simulink model "Week1_problem2"  (R2020b)
settings: Solver=VariableStepAuto  StartTime=0.0  StopTime=100.0  RelTol=1e-3
values from neighbouring files (symbols this model uses):
  b = 50    [parameter_initialize.m]
  k1 = 10    [parameter_initialize.m]
  k2 = 20    [parameter_initialize.m]
  M1 = 100    [parameter_initialize.m]
  M2 = 50    [parameter_initialize.m]
settings Model: Creator=omkar  LastModifiedBy=omkar

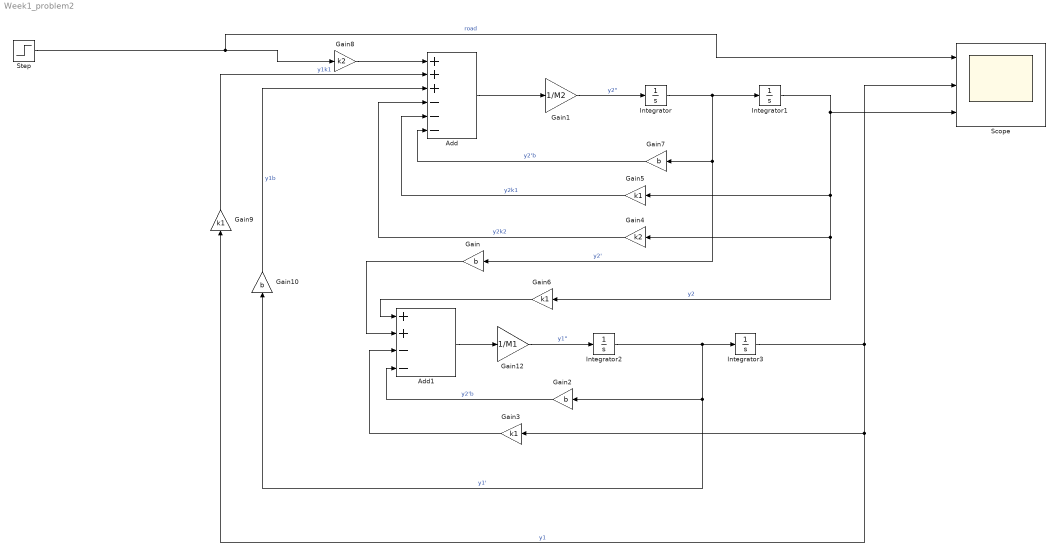
== system Week1_problem2 ==
  Add : Sum  Inputs=+++---
  Add1 : Sum  Inputs=++--
  Gain{,2,7,10} (4 alike) : Gain  Gain=b
  Gain1 : Gain  Gain=1/M2
  Gain12 : Gain  Gain=1/M1
  Gain{3,5..6,9} (4 alike) : Gain  Gain=k1
  Gain4 : Gain  Gain=k2
  Gain8 : Gain  Gain=k2
  Integrator{,1..3} (4 alike) : Integrator
  Scope : Scope  NumInputPorts=3
  Step : Step  SampleTime=0
  wires:
  Add/1 -> Gain1/1
  Gain1/1 -> Integrator/1  "y2\""
  Integrator/1 -> Gain/1, Gain7/1, Integrator1/1  "y2'"
  Gain7/1 -> Add/6  "y2'b"
  Integrator1/1 -> Gain5/1, Gain4/1, Gain6/1, Scope/3  "y2"
  Gain6/1 -> Add1/1
  Gain/1 -> Add1/2
  Add1/1 -> Gain12/1
  Gain12/1 -> Integrator2/1  "y1\""
  Integrator2/1 -> Gain2/1, Gain10/1, Integrator3/1  "y1'"
  Integrator3/1 -> Scope/2, Gain3/1, Gain9/1  "y1"
  Gain2/1 -> Add1/4  "y2'b"
  Gain3/1 -> Add1/3
  Gain5/1 -> Add/5  "y2k1"
  Gain4/1 -> Add/4  "y2k2"
  Gain8/1 -> Add/1
  Gain9/1 -> Add/2  "y1k1"
  Gain10/1 -> Add/3  "y1b"
  Step/1 -> Scope/1, Gain8/1  "road"
